simulink model "gps_model"  (R2020a)
settings: Solver=VariableStepAuto  StartTime=0.0  StopTime=5600  MaxStep=1  MinStep=1  RelTol=1e-3
libraries: simulink x1
settings Model: Creator=lu  LastModifiedBy=utente
settings DataIOCC: ReturnWorkspaceOutputs=off
settings DebuggingCC: ArithmeticOperatorsInVariantConditions=warning
settings SFSimCC: CustomCodeUndefinedFunction=UseInterfaceOnly

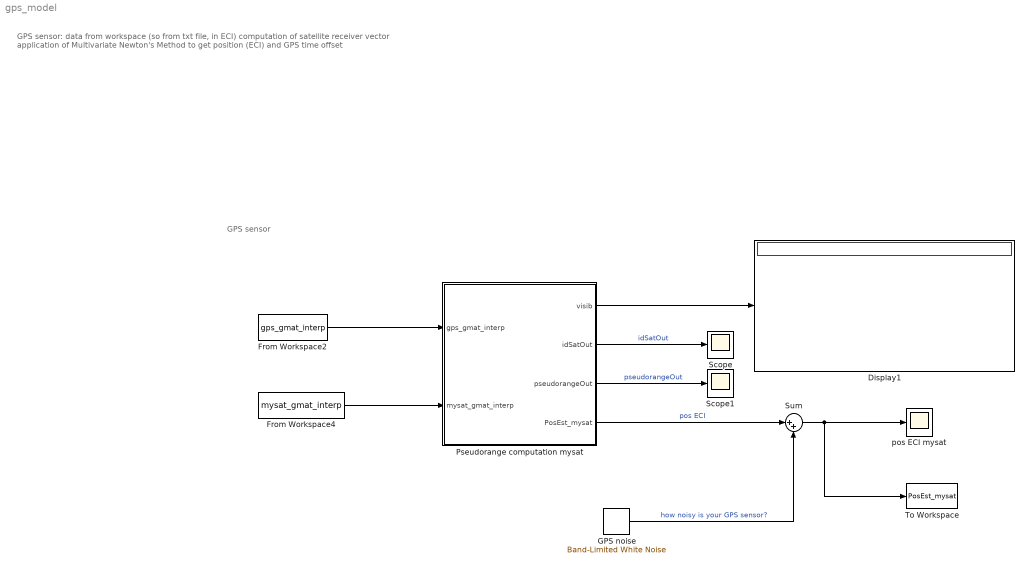
== system gps_model ==
  note: GPS sensor
  note: GPS sensor: data from workspace (so from txt file, in ECI)
      | computation of satellite receiver vector
      | application of Multivariate Newton's Method to get position (ECI) and GPS time offset
  Display1 : Display
  From Workspace2 : FromWorkspace  VariableName=gps_gmat_interp
  From Workspace4 : FromWorkspace  VariableName=mysat_gmat_interp
  GPS noise : simulink/Sources/Band-Limited White Noise  Cov=[0]  Ts=1  seed=[23341]
  Pseudorange computation mysat : MATLAB Function  TreatAsAtomicUnit=on
  Scope : Scope
  Scope1 : Scope
  Sum : Sum  Inputs=|++
  To Workspace : ToWorkspace  VariableName=PosEst_mysat  SaveFormat=Timeseries  SampleTime=-1
  pos ECI mysat : Scope
  wires:
  From Workspace4/1 -> Pseudorange computation mysat/2(mysat_gmat_interp)
  From Workspace2/1 -> Pseudorange computation mysat/1(gps_gmat_interp)
  Pseudorange computation mysat/1(visib) -> Display1/1
  Pseudorange computation mysat/2(idSatOut) -> Scope/1  "idSatOut"
  Pseudorange computation mysat/3(pseudorangeOut) -> Scope1/1  "pseudorangeOut"
  Pseudorange computation mysat/4(PosEst_mysat) -> Sum/1  "pos ECI"
  Sum/1 -> To Workspace/1, pos ECI mysat/1
  GPS noise/1 -> Sum/2  "how noisy is your GPS sensor?"

== matlab function gps_model/Pseudorange computation mysat ==
  data: gps_gmat_interp input; visib output; mysat_gmat_interp input; idSatOut output; pseudorangeOut output; PosEst_mysat output
function [visib, idSatOut, pseudorangeOut, PosEst_mysat]   = fcn(gps_gmat_interp, mysat_gmat_interp)

totsat=24; % satellites in gps constellation
c=299792.458; %speed of light [km/s]

numsat = 0; % number of visible satellite
visib = zeros(1,totsat); % visibility vector
dist = zeros(1,totsat); % distance from gps satellite to mysat
elev = zeros(1,totsat); % gps satellite elevation
pseudorange = zeros(1,totsat); % pseudorange between gps satellite and mysat
idSat = zeros(1,totsat); % identification of gps satellite
tt=zeros(1,totsat); % trasmission time

for satellite = 1:totsat % for each satellite in the gps constellation
    % Extract satellite i position
    posSat = gps_gmat_interp(3*(satellite-1)+1:3*(satellite-1)+3,:);    
    
    % computation of gps satellite receiver vector
    sl = posSat-mysat_gmat_interp;
    dist(satellite) = norm(sl);
    hSat = mysat_gmat_interp'/norm(mysat_gmat_interp)*sl;
    elev(satellite) = asin(hSat/norm(sl));
    
    % visibility of the gps satellite
    if hSat > 0 && elev(satellite) >= 5*pi/180
        visib(satellite) = 1; % is visible
        numsat=numsat+1; % update n° of visible gps satellites
        pseudorange(numsat) = dist(satellite)+10^-3*randi([-50,+50]); % update pseudoranges     
        idSat(numsat) = satellite;
        tt(numsat)=pseudorange(numsat)/c;
    else
        visib(satellite) = 0;
    end
end
idSatOut = idSat(1:4);
pseudorangeOut = pseudorange(1:4);
ttOut=tt(1:4);

%% solution (Multivariate Newton's Method)
% ref: http://mason.gmu.edu/~nulloaso/Project2.html

% position of visible gps satellites (4 sats)
PsatVis = zeros(3,4);
for nsat = 1:4
    PsatVis(:,nsat)=gps_gmat_interp(3*(idSatOut(nsat)-1)+1:3*(idSatOut(nsat)-1)+3);
end

% simultaneous satellite positions [km]
A1= PsatVis(1,1); B1= PsatVis(2,1); C1= PsatVis(3,1);
A2 = PsatVis(1,2); B2= PsatVis(2,2); C2=PsatVis(3,2);
A3 = PsatVis(1,3); B3 = PsatVis(2,3); C3= PsatVis(3,3);
A4= PsatVis(1,4); B4=PsatVis(2,4); C4=PsatVis(3,4);

% trasmission time intervals [s]
t1= ttOut(1);
t2= ttOut(2);
t3= ttOut(3);
t4= ttOut(4);

% initial vector
u= [0;0;6370+400;0]; % [x_eci y_eci z_eci time_delay]

x=zeros(1,10);
y=zeros(1,10);
z=zeros(1,10);
d=zeros(1,10);

% iteration
for i=1: 10
   
    x(i)= u(1);
    y(i)= u(2) ;
    z(i)= u(3);
    d(i)= u(4);
    
    % functions of (x,y,z,d), from (4.73)
    f1= ( x(i)-A1).^2 + (y(i)-B1).^2 + (z(i)-C1).^2 - (c*(t1 - d(i))).^2;
    f2= ( x(i)-A2).^2 + (y(i)-B2).^2 + (z(i)-C2).^2 - (c*(t2 - d(i))).^2;
    f3= ( x(i)-A3).^2 + (y(i)-B3).^2 + (z(i)-C3).^2 - (c*(t3 - d(i))).^2;
    f4= ( x(i)-A4).^2 + (y(i)-B4).^2 + (z(i)-C4).^2 - (c*(t4 - d(i))).^2; 
    F = [f1;f2;f3;f4];
   
   % Jacobian Matrix
   df1x= (2*(x(i)-A1));
   df1y= (2*(y(i)-B1));
   df1z= (2*(z(i)-C1));
   df1t= (2*c^2*(t1-d(i)));
 
   df2x=2*(x(i)-A2);
   df2y=2*(y(i)-B2);
   df2z=2*(z(i)-C2);
   df2t=2*c^2*(t2-d(i));

   df3x=2*(x(i)-A3);
   df3y=2*(y(i)-B3);
   df3z=2*(z(i)-C3);
   df3t=2*c^2*(t3-d(i));

   df4x=2*(x(i)-A4);
   df4y=2*(y(i)-B4);
   df4z=2*(z(i)-C4);
   df4t=2*c^2*(t4-d(i));

   DF = [df1x, df1y, df1z, df1t; df2x, df2y df2z df2t;df3x df3y df3z df3t;df4x df4y df4z df4t];
   
   % new u(x,y,z,d) vector
    V = DF\(-F);
    u = u+V;

end

PosEst_mysat=u;
